simulink model "single_leg_dynamictest"  (R2022a)
settings: Solver=FixedStepAuto  StartTime=0.0  StopTime=20  FixedStep=1e-3  RelTol=1e-3
undefined symbols (not defined in the file or in its folder): X, Y, Z
libraries: sm_lib x46, nesl_utility x13, Contact_Forces_Lib x1
(part 2 of 2)

== matlab function single_leg_dynamictest/Dynamics ==
  data: theta2 input; theta3 input; dtheta1 input; dtheta2 input; dtheta3 input; t1 output; t2 output; t3 output; ddtheta1 input; ddtheta2 input; ddtheta3 input
%function [t1,t2,t3] = fcn(theta1,theta2,theta3,dtheta1,dtheta2,dtheta3,ddtheta1,ddtheta2,ddtheta3)
function [t1,t2,t3] = fcn(theta2,theta3,dtheta1,dtheta2,dtheta3,ddtheta1,ddtheta2,ddtheta3)
m1=2.26887;m2=1.53078;m3=2.26236;
J1x=0.00724219;J1y=0.0160606;J1z=0.018338;
J1yz=0;J1zx=0;J1xy=-0.00117504;
J2x=0.0221893;J2y=0.00165664;J2z=0.0223625;
J2yz=0.000161544;J2zx=0;J2xy=-0.000216533;
J3x=0.0502385;J3y=0.00540476;J3z=0.0526685;
J3yz=-0.000480415;J3zx=-9.45532e-5;J3xy=0.000773023;
L1=0.3;L2=0.27;L3=0.5;
g=9.8;

% t1=(J2x*ddtheta1)/2 + (J3x*ddtheta1)/2 + J1y*ddtheta1 + (J2y*ddtheta1)/2 + (J3y*ddtheta1)/2 + (71742288219087375296683149304729*ddtheta1*m1)/5192296858534827628530496329220096 + (224915364647171551817573576679381139*ddtheta1*m2)/42535295865117307932921825928971026432 + (110003100955735299101016157360209849*ddtheta1*m3)/5316911983139663491615228241121378304 - (41229240673166744905400286918375*ddtheta2*m2*cos(theta2))/21267647932558653966460912964485513216 + (32413724259249712723599481432425*ddtheta2*m2*sin(theta2))/166153499473114484112975882535043072 - J3yz*dtheta2^2*cos(theta2 + theta3) - J3yz*dtheta3^2*cos(theta2 + theta3) + J3zx*dtheta2^2*sin(theta2 + theta3) + J3zx*dtheta3^2*sin(theta2 + theta3) + (11303477583825805338660830691353*dtheta2^2*m3*cos(theta2 + theta3))/20769187434139310514121985316880384 + (11303477583825805338660830691353*dtheta3^2*m3*cos(theta2 + theta3))/20769187434139310514121985316880384 + (J2x*ddtheta1*cos(2*theta2))/2 - (J2y*ddtheta1*cos(2*theta2))/2 - J2yz*dtheta2^2*cos(theta2) - (52091429297631985777908461222871*dtheta2^2*m3*sin(theta2 + theta3))/332306998946228968225951765070086144 - (52091429297631985777908461222871*dtheta3^2*m3*sin(theta2 + theta3))/332306998946228968225951765070086144 - J2xy*ddtheta1*sin(2*theta2) - J2zx*dtheta2^2*sin(theta2) + (224717789977006155621391351965393839*ddtheta1*m2*cos(2*theta2))/42535295865117307932921825928971026432 + (32413724259249712723599481432425*dtheta2^2*m2*cos(theta2))/166153499473114484112975882535043072 + (17447644634598216827789536101855*ddtheta1*m2*sin(2*theta2))/166153499473114484112975882535043072 + (41229240673166744905400286918375*dtheta2^2*m2*sin(theta2))/21267647932558653966460912964485513216 + (J3x*ddtheta1*cos(2*theta2 + 2*theta3))/2 - (J3y*ddtheta1*cos(2*theta2 + 2*theta3))/2 + J3xy*ddtheta1*sin(2*theta2 + 2*theta3) + (727458219877961487502491402943207*ddtheta1*m3*cos(2*theta2 + 2*theta3))/41538374868278621028243970633760768 - (14280189767105151140366067830007*ddtheta1*m3*sin(2*theta2 + 2*theta3))/1298074214633706907132624082305024 - J3zx*ddtheta2*cos(theta2 + theta3) - J3zx*ddtheta3*cos(theta2 + theta3) - J3yz*ddtheta2*sin(theta2 + theta3) - J3yz*ddtheta3*sin(theta2 + theta3) + L1^2*ddtheta1*m2 + L1^2*ddtheta1*m3 + (L2^2*ddtheta1*m3)/2 + (52091429297631985777908461222871*ddtheta2*m3*cos(theta2 + theta3))/332306998946228968225951765070086144 + (52091429297631985777908461222871*ddtheta3*m3*cos(theta2 + theta3))/332306998946228968225951765070086144 + J2zx*ddtheta2*cos(theta2) + (11303477583825805338660830691353*ddtheta2*m3*sin(theta2 + theta3))/20769187434139310514121985316880384 + (11303477583825805338660830691353*ddtheta3*m3*sin(theta2 + theta3))/20769187434139310514121985316880384 - J2yz*ddtheta2*sin(theta2) - (727458219877961487502491402943207*dtheta1*dtheta2*m3*sin(2*theta2 + 2*theta3))/20769187434139310514121985316880384 - (727458219877961487502491402943207*dtheta1*dtheta3*m3*sin(2*theta2 + 2*theta3))/20769187434139310514121985316880384 + (L2^2*ddtheta1*m3*cos(2*theta2))/2 - 2*J3yz*dtheta2*dtheta3*cos(theta2 + theta3) + (1760312979151051*L1*ddtheta1*m3*cos(theta2 + theta3))/4503599627370496 + 2*J3zx*dtheta2*dtheta3*sin(theta2 + theta3) - (8112301582865157*L1*ddtheta1*m3*sin(theta2 + theta3))/72057594037927936 + (11303477583825805338660830691353*dtheta2*dtheta3*m3*cos(theta2 + theta3))/10384593717069655257060992658440192 - (52091429297631985777908461222871*dtheta2*dtheta3*m3*sin(theta2 + theta3))/166153499473114484112975882535043072 + (3703652247158439*L1*ddtheta1*m2*cos(theta2))/18014398509481984 + (1760312979151051*L2*ddtheta1*m3*cos(theta3))/9007199254740992 + (4710929501543945*L1*ddtheta1*m2*sin(theta2))/2305843009213693952 - (8112301582865157*L2*ddtheta1*m3*sin(theta3))/144115188075855872 + (6421288553628203*L2*ddtheta2*m3*sin(theta2))/2305843009213693952 + (1760312979151051*L2*ddtheta1*m3*cos(2*theta2 + theta3))/9007199254740992 - (8112301582865157*L2*ddtheta1*m3*sin(2*theta2 + theta3))/144115188075855872 - 2*J2xy*dtheta1*dtheta2*cos(2*theta2) + (6421288553628203*L2*dtheta2^2*m3*cos(theta2))/2305843009213693952 - J2x*dtheta1*dtheta2*sin(2*theta2) + J2y*dtheta1*dtheta2*sin(2*theta2) + (17447644634598216827789536101855*dtheta1*dtheta2*m2*cos(2*theta2))/83076749736557242056487941267521536 - (224717789977006155621391351965393839*dtheta1*dtheta2*m2*sin(2*theta2))/21267647932558653966460912964485513216 + 2*J3xy*dtheta1*dtheta2*cos(2*theta2 + 2*theta3) + 2*J3xy*dtheta1*dtheta3*cos(2*theta2 + 2*theta3) - J3x*dtheta1*dtheta2*sin(2*theta2 + 2*theta3) - J3x*dtheta1*dtheta3*sin(2*theta2 + 2*theta3) + J3y*dtheta1*dtheta2*sin(2*theta2 + 2*theta3) + J3y*dtheta1*dtheta3*sin(2*theta2 + 2*theta3) - (14280189767105151140366067830007*dtheta1*dtheta2*m3*cos(2*theta2 + 2*theta3))/649037107316853453566312041152512 - (14280189767105151140366067830007*dtheta1*dtheta3*m3*cos(2*theta2 + 2*theta3))/649037107316853453566312041152512 - L2^2*dtheta1*dtheta2*m3*sin(2*theta2) - (8112301582865157*L1*dtheta1*dtheta2*m3*cos(theta2 + theta3))/72057594037927936 - (8112301582865157*L1*dtheta1*dtheta3*m3*cos(theta2 + theta3))/72057594037927936 - (1760312979151051*L1*dtheta1*dtheta2*m3*sin(theta2 + theta3))/4503599627370496 - (1760312979151051*L1*dtheta1*dtheta3*m3*sin(theta2 + theta3))/4503599627370496 + 2*L1*L2*ddtheta1*m3*cos(theta2) + (4710929501543945*L1*dtheta1*dtheta2*m2*cos(theta2))/2305843009213693952 - (8112301582865157*L2*dtheta1*dtheta3*m3*cos(theta3))/144115188075855872 - (3703652247158439*L1*dtheta1*dtheta2*m2*sin(theta2))/18014398509481984 - (1760312979151051*L2*dtheta1*dtheta3*m3*sin(theta3))/9007199254740992 - (8112301582865157*L2*dtheta1*dtheta2*m3*cos(2*theta2 + theta3))/72057594037927936 - (8112301582865157*L2*dtheta1*dtheta3*m3*cos(2*theta2 + theta3))/144115188075855872 - (1760312979151051*L2*dtheta1*dtheta2*m3*sin(2*theta2 + theta3))/4503599627370496 - (1760312979151051*L2*dtheta1*dtheta3*m3*sin(2*theta2 + theta3))/9007199254740992 - 2*L1*L2*dtheta1*dtheta2*m3*sin(theta2);
% t2=J2z*ddtheta2 + J3z*ddtheta2 + J3z*ddtheta3 + (224762175690543189785583629497719889*ddtheta2*m2)/21267647932558653966460912964485513216 + (859077093820674550951101892212505*ddtheta2*m3)/20769187434139310514121985316880384 + (859077093820674550951101892212505*ddtheta3*m3)/20769187434139310514121985316880384 - (41229240673166744905400286918375*ddtheta1*m2*cos(theta2))/21267647932558653966460912964485513216 + (727458219877961487502491402943207*dtheta1^2*m3*sin(2*theta2 + 2*theta3))/41538374868278621028243970633760768 + (3703652247158439*g*m2*cos(theta2))/36028797018963968 + (32413724259249712723599481432425*ddtheta1*m2*sin(theta2))/166153499473114484112975882535043072 + (4710929501543945*g*m2*sin(theta2))/4611686018427387904 + J2xy*dtheta1^2*cos(2*theta2) + (J2x*dtheta1^2*sin(2*theta2))/2 - (J2y*dtheta1^2*sin(2*theta2))/2 - J3zx*ddtheta1*cos(theta2 + theta3) - (17447644634598216827789536101855*dtheta1^2*m2*cos(2*theta2))/166153499473114484112975882535043072 - J3yz*ddtheta1*sin(theta2 + theta3) + (224717789977006155621391351965393839*dtheta1^2*m2*sin(2*theta2))/42535295865117307932921825928971026432 - J3xy*dtheta1^2*cos(2*theta2 + 2*theta3) + L2^2*ddtheta2*m3 + (52091429297631985777908461222871*ddtheta1*m3*cos(theta2 + theta3))/332306998946228968225951765070086144 + (1760312979151051*g*m3*cos(theta2 + theta3))/9007199254740992 + J2zx*ddtheta1*cos(theta2) + (J3x*dtheta1^2*sin(2*theta2 + 2*theta3))/2 - (J3y*dtheta1^2*sin(2*theta2 + 2*theta3))/2 + (11303477583825805338660830691353*ddtheta1*m3*sin(theta2 + theta3))/20769187434139310514121985316880384 - (8112301582865157*g*m3*sin(theta2 + theta3))/144115188075855872 - J2yz*ddtheta1*sin(theta2) + (14280189767105151140366067830007*dtheta1^2*m3*cos(2*theta2 + 2*theta3))/1298074214633706907132624082305024 + (1760312979151051*L2*ddtheta2*m3*cos(theta3))/4503599627370496 + (1760312979151051*L2*ddtheta3*m3*cos(theta3))/9007199254740992 + L2*g*m3*cos(theta2) + (6421288553628203*L2*ddtheta1*m3*sin(theta2))/2305843009213693952 - (8112301582865157*L2*ddtheta2*m3*sin(theta3))/72057594037927936 - (8112301582865157*L2*ddtheta3*m3*sin(theta3))/144115188075855872 + (L2^2*dtheta1^2*m3*sin(2*theta2))/2 + (8112301582865157*L1*dtheta1^2*m3*cos(theta2 + theta3))/144115188075855872 + (1760312979151051*L1*dtheta1^2*m3*sin(theta2 + theta3))/9007199254740992 - (4710929501543945*L1*dtheta1^2*m2*cos(theta2))/4611686018427387904 - (8112301582865157*L2*dtheta3^2*m3*cos(theta3))/144115188075855872 + (3703652247158439*L1*dtheta1^2*m2*sin(theta2))/36028797018963968 - (1760312979151051*L2*dtheta3^2*m3*sin(theta3))/9007199254740992 + (8112301582865157*L2*dtheta1^2*m3*cos(2*theta2 + theta3))/144115188075855872 + (1760312979151051*L2*dtheta1^2*m3*sin(2*theta2 + theta3))/9007199254740992 + L1*L2*dtheta1^2*m3*sin(theta2) - (8112301582865157*L2*dtheta2*dtheta3*m3*cos(theta3))/72057594037927936 - (1760312979151051*L2*dtheta2*dtheta3*m3*sin(theta3))/4503599627370496;
% t3=J3z*ddtheta2 + J3z*ddtheta3 + (859077093820674550951101892212505*ddtheta2*m3)/20769187434139310514121985316880384 + (859077093820674550951101892212505*ddtheta3*m3)/20769187434139310514121985316880384 + (727458219877961487502491402943207*dtheta1^2*m3*sin(2*theta2 + 2*theta3))/41538374868278621028243970633760768 - J3zx*ddtheta1*cos(theta2 + theta3) - J3yz*ddtheta1*sin(theta2 + theta3) - J3xy*dtheta1^2*cos(2*theta2 + 2*theta3) + (52091429297631985777908461222871*ddtheta1*m3*cos(theta2 + theta3))/332306998946228968225951765070086144 + (1760312979151051*g*m3*cos(theta2 + theta3))/9007199254740992 + (J3x*dtheta1^2*sin(2*theta2 + 2*theta3))/2 - (J3y*dtheta1^2*sin(2*theta2 + 2*theta3))/2 + (11303477583825805338660830691353*ddtheta1*m3*sin(theta2 + theta3))/20769187434139310514121985316880384 - (8112301582865157*g*m3*sin(theta2 + theta3))/144115188075855872 + (14280189767105151140366067830007*dtheta1^2*m3*cos(2*theta2 + 2*theta3))/1298074214633706907132624082305024 + (1760312979151051*L2*ddtheta2*m3*cos(theta3))/9007199254740992 - (8112301582865157*L2*ddtheta2*m3*sin(theta3))/144115188075855872 + (8112301582865157*L1*dtheta1^2*m3*cos(theta2 + theta3))/144115188075855872 + (1760312979151051*L1*dtheta1^2*m3*sin(theta2 + theta3))/9007199254740992 + (8112301582865157*L2*dtheta1^2*m3*cos(theta3))/288230376151711744 + (8112301582865157*L2*dtheta2^2*m3*cos(theta3))/144115188075855872 + (1760312979151051*L2*dtheta1^2*m3*sin(theta3))/18014398509481984 + (1760312979151051*L2*dtheta2^2*m3*sin(theta3))/9007199254740992 + (8112301582865157*L2*dtheta1^2*m3*cos(2*theta2 + theta3))/288230376151711744 + (1760312979151051*L2*dtheta1^2*m3*sin(2*theta2 + theta3))/18014398509481984;
%t1=ddtheta1*(J1y + 0.0138*m1);
%重力补偿项
%t1=0;
%t2=(g*(0.1954*m3*cos(theta2 + theta3) - 0.0563*m3*sin(theta2 + theta3) + 0.1028*m2*cos(theta2) + L2*m3*cos(theta2)));
%t3=(g*m3*(28165007666416816*cos(theta2 + theta3) - 8112301582865157*sin(theta2 + theta3)))/144115188075855872;
%t3=t3+J3z*ddtheta2 + J3z*ddtheta3 + 0.04136*ddtheta2*m3 + 0.04136*ddtheta3*m3 - J3xy*dtheta1^2*cos(2.0*theta2 + 2.0*theta3) + 0.5*J3x*dtheta1^2*sin(2.0*theta2 + 2.0*theta3) - 0.5*J3y*dtheta1^2*sin(2.0*theta2 + 2.0*theta3) + 0.011001058033599999297657186936306*dtheta1^2*m3*cos(2.0*theta2 + 2.0*theta3) + 0.017512919611919999484960694431379*dtheta1^2*m3*sin(2.0*theta2 + 2.0*theta3) - 1.0*J3zx*ddtheta1*cos(theta2 + theta3) - 1.0*J3yz*ddtheta1*sin(theta2 + theta3) + 0.00015675694301599999806692144233011*ddtheta1*m3*cos(theta2 + theta3)  + 0.00054424264886000000915784662103292*ddtheta1*m3*sin(theta2 + theta3) + 0.02814519999999999869122468965088*L2*dtheta1^2*m3*cos(2.0*theta2 + theta3) + 0.097716999999999998305355575212161*L2*dtheta1^2*m3*sin(2.0*theta2 + theta3) + 0.19543399999999999661071115042432*L2*ddtheta2*m3*cos(theta3) - 0.056290399999999997382449379301761*L2*ddtheta2*m3*sin(theta3) + 0.056290399999999997382449379301761*L1*dtheta1^2*m3*cos(theta2 + theta3) + 0.19543399999999999661071115042432*L1*dtheta1^2*m3*sin(theta2 + theta3) + 0.02814519999999999869122468965088*L2*dtheta1^2*m3*cos(theta3) + 0.056290399999999997382449379301761*L2*dtheta2^2*m3*cos(theta3) + 0.097716999999999998305355575212161*L2*dtheta1^2*m3*sin(theta3) + 0.19543399999999999661071115042432*L2*dtheta2^2*m3*sin(theta3);
t1=(J2x*ddtheta1)/2 + (J3x*ddtheta1)/2 + J1y*ddtheta1 + (J2y*ddtheta1)/2 + (J3y*ddtheta1)/2 + (71742288219087375296683149304729*ddtheta1*m1)/5192296858534827628530496329220096 + (13717039967881754925749968916721*ddtheta1*m2)/2596148429267413814265248164610048 + (110003100955735299101016157360209849*ddtheta1*m3)/5316911983139663491615228241121378304 - J3yz*dtheta2^2*cos(theta2 + theta3) - J3yz*dtheta3^2*cos(theta2 + theta3) + J3zx*dtheta2^2*sin(theta2 + theta3) + J3zx*dtheta3^2*sin(theta2 + theta3) + (11303477583825805338660830691353*dtheta2^2*m3*cos(theta2 + theta3))/20769187434139310514121985316880384 + (11303477583825805338660830691353*dtheta3^2*m3*cos(theta2 + theta3))/20769187434139310514121985316880384 + (J2x*ddtheta1*cos(2*theta2))/2 - (J2y*ddtheta1*cos(2*theta2))/2 - J2yz*dtheta2^2*cos(theta2) - (52091429297631985777908461222871*dtheta2^2*m3*sin(theta2 + theta3))/332306998946228968225951765070086144 - (52091429297631985777908461222871*dtheta3^2*m3*sin(theta2 + theta3))/332306998946228968225951765070086144 - J2xy*ddtheta1*sin(2*theta2) - J2zx*dtheta2^2*sin(theta2) + (13717039967881754925749968916721*ddtheta1*m2*cos(2*theta2))/2596148429267413814265248164610048 + (J3x*ddtheta1*cos(2*theta2 + 2*theta3))/2 - (J3y*ddtheta1*cos(2*theta2 + 2*theta3))/2 + J3xy*ddtheta1*sin(2*theta2 + 2*theta3) + (727458219877961487502491402943207*ddtheta1*m3*cos(2*theta2 + 2*theta3))/41538374868278621028243970633760768 - (14280189767105151140366067830007*ddtheta1*m3*sin(2*theta2 + 2*theta3))/1298074214633706907132624082305024 - J3zx*ddtheta2*cos(theta2 + theta3) - J3zx*ddtheta3*cos(theta2 + theta3) - J3yz*ddtheta2*sin(theta2 + theta3) - J3yz*ddtheta3*sin(theta2 + theta3) + L1^2*ddtheta1*m2 + L1^2*ddtheta1*m3 + (L2^2*ddtheta1*m3)/2 + (52091429297631985777908461222871*ddtheta2*m3*cos(theta2 + theta3))/332306998946228968225951765070086144 + (52091429297631985777908461222871*ddtheta3*m3*cos(theta2 + theta3))/332306998946228968225951765070086144 + J2zx*ddtheta2*cos(theta2) + (11303477583825805338660830691353*ddtheta2*m3*sin(theta2 + theta3))/20769187434139310514121985316880384 + (11303477583825805338660830691353*ddtheta3*m3*sin(theta2 + theta3))/20769187434139310514121985316880384 - J2yz*ddtheta2*sin(theta2) - (727458219877961487502491402943207*dtheta1*dtheta2*m3*sin(2*theta2 + 2*theta3))/20769187434139310514121985316880384 - (727458219877961487502491402943207*dtheta1*dtheta3*m3*sin(2*theta2 + 2*theta3))/20769187434139310514121985316880384 + (L2^2*ddtheta1*m3*cos(2*theta2))/2 - 2*J3yz*dtheta2*dtheta3*cos(theta2 + theta3) + (1760312979151051*L1*ddtheta1*m3*cos(theta2 + theta3))/4503599627370496 + 2*J3zx*dtheta2*dtheta3*sin(theta2 + theta3) - (8112301582865157*L1*ddtheta1*m3*sin(theta2 + theta3))/72057594037927936 + (11303477583825805338660830691353*dtheta2*dtheta3*m3*cos(theta2 + theta3))/10384593717069655257060992658440192 - (52091429297631985777908461222871*dtheta2*dtheta3*m3*sin(theta2 + theta3))/166153499473114484112975882535043072 + (3703652247158439*L1*ddtheta1*m2*cos(theta2))/18014398509481984 + (1760312979151051*L2*ddtheta1*m3*cos(theta3))/9007199254740992 - (8112301582865157*L2*ddtheta1*m3*sin(theta3))/144115188075855872 + (6421288553628203*L2*ddtheta2*m3*sin(theta2))/2305843009213693952 + (1760312979151051*L2*ddtheta1*m3*cos(2*theta2 + theta3))/9007199254740992 - (8112301582865157*L2*ddtheta1*m3*sin(2*theta2 + theta3))/144115188075855872 - 2*J2xy*dtheta1*dtheta2*cos(2*theta2) + (6421288553628203*L2*dtheta2^2*m3*cos(theta2))/2305843009213693952 - J2x*dtheta1*dtheta2*sin(2*theta2) + J2y*dtheta1*dtheta2*sin(2*theta2) - (13717039967881754925749968916721*dtheta1*dtheta2*m2*sin(2*theta2))/1298074214633706907132624082305024 + 2*J3xy*dtheta1*dtheta2*cos(2*theta2 + 2*theta3) + 2*J3xy*dtheta1*dtheta3*cos(2*theta2 + 2*theta3) - J3x*dtheta1*dtheta2*sin(2*theta2 + 2*theta3) - J3x*dtheta1*dtheta3*sin(2*theta2 + 2*theta3) + J3y*dtheta1*dtheta2*sin(2*theta2 + 2*theta3) + J3y*dtheta1*dtheta3*sin(2*theta2 + 2*theta3) - (14280189767105151140366067830007*dtheta1*dtheta2*m3*cos(2*theta2 + 2*theta3))/649037107316853453566312041152512 - (14280189767105151140366067830007*dtheta1*dtheta3*m3*cos(2*theta2 + 2*theta3))/649037107316853453566312041152512 - L2^2*dtheta1*dtheta2*m3*sin(2*theta2) - (8112301582865157*L1*dtheta1*dtheta2*m3*cos(theta2 + theta3))/72057594037927936 - (8112301582865157*L1*dtheta1*dtheta3*m3*cos(theta2 + theta3))/72057594037927936 - (1760312979151051*L1*dtheta1*dtheta2*m3*sin(theta2 + theta3))/4503599627370496 - (1760312979151051*L1*dtheta1*dtheta3*m3*sin(theta2 + theta3))/4503599627370496 + 2*L1*L2*ddtheta1*m3*cos(theta2) - (8112301582865157*L2*dtheta1*dtheta3*m3*cos(theta3))/144115188075855872 - (3703652247158439*L1*dtheta1*dtheta2*m2*sin(theta2))/18014398509481984 - (1760312979151051*L2*dtheta1*dtheta3*m3*sin(theta3))/9007199254740992 - (8112301582865157*L2*dtheta1*dtheta2*m3*cos(2*theta2 + theta3))/72057594037927936 - (8112301582865157*L2*dtheta1*dtheta3*m3*cos(2*theta2 + theta3))/144115188075855872 - (1760312979151051*L2*dtheta1*dtheta2*m3*sin(2*theta2 + theta3))/4503599627370496 - (1760312979151051*L2*dtheta1*dtheta3*m3*sin(2*theta2 + theta3))/9007199254740992 - 2*L1*L2*dtheta1*dtheta2*m3*sin(theta2);
t2=J2z*ddtheta2 + J3z*ddtheta2 + J3z*ddtheta3 + (13717039967881754925749968916721*ddtheta2*m2)/1298074214633706907132624082305024 + (859077093820674550951101892212505*ddtheta2*m3)/20769187434139310514121985316880384 + (859077093820674550951101892212505*ddtheta3*m3)/20769187434139310514121985316880384 + (727458219877961487502491402943207*dtheta1^2*m3*sin(2*theta2 + 2*theta3))/41538374868278621028243970633760768 + (3703652247158439*g*m2*cos(theta2))/36028797018963968 + J2xy*dtheta1^2*cos(2*theta2) + (J2x*dtheta1^2*sin(2*theta2))/2 - (J2y*dtheta1^2*sin(2*theta2))/2 - J3zx*ddtheta1*cos(theta2 + theta3) - J3yz*ddtheta1*sin(theta2 + theta3) + (13717039967881754925749968916721*dtheta1^2*m2*sin(2*theta2))/2596148429267413814265248164610048 - J3xy*dtheta1^2*cos(2*theta2 + 2*theta3) + L2^2*ddtheta2*m3 + (52091429297631985777908461222871*ddtheta1*m3*cos(theta2 + theta3))/332306998946228968225951765070086144 + (1760312979151051*g*m3*cos(theta2 + theta3))/9007199254740992 + J2zx*ddtheta1*cos(theta2) + (J3x*dtheta1^2*sin(2*theta2 + 2*theta3))/2 - (J3y*dtheta1^2*sin(2*theta2 + 2*theta3))/2 + (11303477583825805338660830691353*ddtheta1*m3*sin(theta2 + theta3))/20769187434139310514121985316880384 - (8112301582865157*g*m3*sin(theta2 + theta3))/144115188075855872 - J2yz*ddtheta1*sin(theta2) + (14280189767105151140366067830007*dtheta1^2*m3*cos(2*theta2 + 2*theta3))/1298074214633706907132624082305024 + (1760312979151051*L2*ddtheta2*m3*cos(theta3))/4503599627370496 + (1760312979151051*L2*ddtheta3*m3*cos(theta3))/9007199254740992 + L2*g*m3*cos(theta2) + (6421288553628203*L2*ddtheta1*m3*sin(theta2))/2305843009213693952 - (8112301582865157*L2*ddtheta2*m3*sin(theta3))/72057594037927936 - (8112301582865157*L2*ddtheta3*m3*sin(theta3))/144115188075855872 + (L2^2*dtheta1^2*m3*sin(2*theta2))/2 + (8112301582865157*L1*dtheta1^2*m3*cos(theta2 + theta3))/144115188075855872 + (1760312979151051*L1*dtheta1^2*m3*sin(theta2 + theta3))/9007199254740992 - (8112301582865157*L2*dtheta3^2*m3*cos(theta3))/144115188075855872 + (3703652247158439*L1*dtheta1^2*m2*sin(theta2))/36028797018963968 - (1760312979151051*L2*dtheta3^2*m3*sin(theta3))/9007199254740992 + (8112301582865157*L2*dtheta1^2*m3*cos(2*theta2 + theta3))/144115188075855872 + (1760312979151051*L2*dtheta1^2*m3*sin(2*theta2 + theta3))/9007199254740992 + L1*L2*dtheta1^2*m3*sin(theta2) - (8112301582865157*L2*dtheta2*dtheta3*m3*cos(theta3))/72057594037927936 - (1760312979151051*L2*dtheta2*dtheta3*m3*sin(theta3))/4503599627370496;
t3=J3z*ddtheta2 + J3z*ddtheta3 + (859077093820674550951101892212505*ddtheta2*m3)/20769187434139310514121985316880384 + (859077093820674550951101892212505*ddtheta3*m3)/20769187434139310514121985316880384 + (727458219877961487502491402943207*dtheta1^2*m3*sin(2*theta2 + 2*theta3))/41538374868278621028243970633760768 - J3zx*ddtheta1*cos(theta2 + theta3) - J3yz*ddtheta1*sin(theta2 + theta3) - J3xy*dtheta1^2*cos(2*theta2 + 2*theta3) + (52091429297631985777908461222871*ddtheta1*m3*cos(theta2 + theta3))/332306998946228968225951765070086144 + (1760312979151051*g*m3*cos(theta2 + theta3))/9007199254740992 + (J3x*dtheta1^2*sin(2*theta2 + 2*theta3))/2 - (J3y*dtheta1^2*sin(2*theta2 + 2*theta3))/2 + (11303477583825805338660830691353*ddtheta1*m3*sin(theta2 + theta3))/20769187434139310514121985316880384 - (8112301582865157*g*m3*sin(theta2 + theta3))/144115188075855872 + (14280189767105151140366067830007*dtheta1^2*m3*cos(2*theta2 + 2*theta3))/1298074214633706907132624082305024 + (1760312979151051*L2*ddtheta2*m3*cos(theta3))/9007199254740992 - (8112301582865157*L2*ddtheta2*m3*sin(theta3))/144115188075855872 + (8112301582865157*L1*dtheta1^2*m3*cos(theta2 + theta3))/144115188075855872 + (1760312979151051*L1*dtheta1^2*m3*sin(theta2 + theta3))/9007199254740992 + (8112301582865157*L2*dtheta1^2*m3*cos(theta3))/288230376151711744 + (8112301582865157*L2*dtheta2^2*m3*cos(theta3))/144115188075855872 + (1760312979151051*L2*dtheta1^2*m3*sin(theta3))/18014398509481984 + (1760312979151051*L2*dtheta2^2*m3*sin(theta3))/9007199254740992 + (8112301582865157*L2*dtheta1^2*m3*cos(2*theta2 + theta3))/288230376151711744 + (1760312979151051*L2*dtheta1^2*m3*sin(2*theta2 + theta3))/18014398509481984;

== matlab function single_leg_dynamictest/cpg.zip/MATLAB Function ==
  data: theta1 input; theta2 input; x output; theta3 input; y output; z output
function [x,y,z] = Forward_Kinematics(theta1,theta2,theta3)
l1=300;
l2=270;
l3=500;

L=l1+l2*cos(theta2)+l3*cos(theta2+theta3);
z=l2*sin(theta2)+l3*sin(theta2+theta3);
x=L*cos(theta1);
y=L*sin(theta1);

== matlab function single_leg_dynamictest/cpg.zip/MATLAB Function1 ==
  data: xp input; yp input; xfd output; zp input; yfd output; zfd output; dxfd output; dyfd output; dzfd output; Step_time input
function [xfd,yfd,zfd,dxfd,dyfd,dzfd] = CPG(xp,yp,zp,Step_time)
alpha=50; %调整足端轨迹收敛到极限环的速度的参数
beta=50; %调整足端轨迹收敛到极限环的速度的参数
Ls=100; %迈步步长
Hs=50; %最大抬腿高度
Vf=100; %期望的机身前进速度
Df=0.1; %占地系数
bp=1.5; %CPG参数，可以修改摆动相和支撑相的切换速度
Kc=10;%半椭圆补偿参数
ztd=-0.5;%触地深度

%足端轨迹坐标系相对于参考坐标系坐标
xp0=0;
yp0=300;
zp0=-230;


%Step_time=0.001; %仿真步长
%simulation_time=10; %仿真总时间

xf=xp;
yf=0;
zf=zp;


if xp==xp0&&zp==zp0
    xp=xp+0.001;
    xf=xf+0.001;
end
x_average=xp-xp0;
z_average=zp-zp0;

ws=pi*(Vf/Ls)*( (Df/(1-Df))*( (exp(-bp*z_average)+1)^-1 ) + (exp(bp*z_average)+1)^-1);

d_xp=(alpha*(1-(4*x_average^2)/(Ls^2)-(z_average^2)/(Hs^2))*x_average+((ws*Ls)/(2*Hs))*z_average)*Step_time;
d_zp=(beta*(1-(4*x_average^2)/(Ls^2)-(z_average^2)/(Hs^2))*z_average-(ws*2*Hs/Ls)*x_average)*Step_time;

xp=xp+d_xp;
zp=zp+d_zp;

d_xf=((( (d_xp/Step_time)+Kc*(xp-xf) )*( exp(-bp*(z_average-ztd))+1)^-1)-Vf*(exp(bp*(z_average-ztd))+1)^-1)*Step_time;
d_zf=((( (d_zp/Step_time)+Kc*(zp-zf) )*( exp(-bp*(z_average-ztd))+1)^-1))*Step_time;
xfd=xf+d_xf;
zfd=zf+d_zf;
yfd=yp;
dxfd=d_xf/Step_time;
dzfd=d_zf/Step_time;
dyfd=0;

== matlab function single_leg_dynamictest/腿1足端轨迹规划 ==
  data: x output; t input; y output; z output
function [x,y,z] = fcn(t)
%半圆足端轨迹规划
r=150;
T=0.5;
t=mod(t,T);
d=0.5;%占空比
Tswing=d*T;
Tstand=(1-d)*T;
if t>=0&&t<=Tswing
    theta=pi/Tswing*t;
    y=r*cos(pi-theta);
    z=r*sin(pi-theta)-300;
else
    z=-300;
    y=r-2*r*(t-Tswing)/Tstand;
end
x=500;
